simulink model "Assignment2 fake"  (R2020a)
settings: Solver=FixedStepAuto  StartTime=0.0  StopTime=10.0  FixedStep=1e-3  RelTol=1e-3  EnableMultiTasking=on
undefined symbols (not defined in the file): A0, A1, D0, D1, D10, D11, D12, D13, D2, D3, D4, D5, D6, D7, D8, D9, PTA0, PTA1, PTA2, PTB2, PTB23, PTB3, PTB9, PTC16, PTC17, PTC2, PTC3, PTC4, PTD0, PTD1, PTD2, PTD3
libraries: frdmk64flib x25, etargetslib x2
settings Model: ExtModeTrigDuration=5  Creator=theodor  LastModifiedBy=theodor
settings OptimizationCC: EnhancedBackFolding=on  PassReuseOutputArgsAs=Individual arguments  ZeroExternalMemoryAtStartup=off  ZeroInternalMemoryAtStartup=off  MaxStackSize=64  OptimizeBlockOrder=speed  DifferentSizesBufferReuse=on  OptimizationCustomize=off  EfficientTunableParamExpr=on
settings DebuggingCC: ParameterTunabilityLossMsg=error
settings HardwareCC: ProdBitPerPointer=32  ProdBitPerSizeT=32  ProdBitPerPtrDiffT=32  ProdLargestAtomicInteger=Long  ProdLargestAtomicFloat=Double  ProdWordSize=32  ProdHWDeviceType=ARM Compatible->ARM Cortex
settings SFSimCC: MATLABDynamicMemAlloc=off
settings RTWCC: SystemTargetFile=ert.tlc  HardwareBoard=NXP FRDM-K64F  TemplateMakefile=ert_default_tmf  Toolchain=GNU Tools for ARM Embedded Processors
settings CodeAppCC: ForceParamTrailComments=on  IgnoreCustomStorageClasses=off  OperatorAnnotations=on  SimulinkDataObjDesc=on  SFDataObjDesc=on  InsertBlockDesc=on

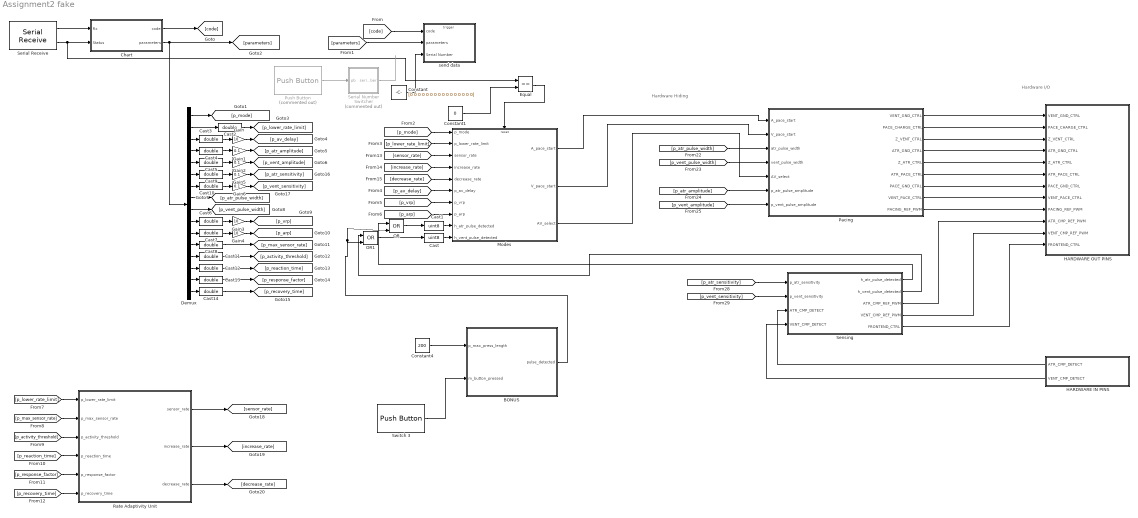
== system Assignment2 fake ==
  note: Hardware I/O
  note: Hardware Hiding
  BONUS : Stateflow chart  TreatAsAtomicUnit=on
  Cast : DataTypeConversion  OutDataTypeStr=uint8
  Cast1 : DataTypeConversion  OutDataTypeStr=uint8
  Cast{2..14} (13 alike) : DataTypeConversion  OutDataTypeStr=double
  Chart : Stateflow chart  TreatAsAtomicUnit=on
  Constant : Constant  Value=[0 0 0 0 0 0 0 0 0 0 0 0 0 0 0 0]  OutDataTypeStr=uint8
  Constant1 : Constant  Value=0
  Constant4 : Constant  Value=200
  Demux : Demux  Outputs=16
  Equal : RelationalOperator  Operator===  OutDataTypeStr=boolean  RndMeth=Simplest
  Gain : Gain  Gain=10
  Gain{1..2,5..6} (4 alike) : Gain  Gain=0.1
  Gain3 : Gain  Gain=10
  Gain4 : Gain  Gain=10
  HARDWARE IN PINS : Subsystem
  HARDWARE OUT PINS : Subsystem
  Modes : Subsystem
  OR : Logic  Operator=OR  IconShape=distinctive  AllPortsSameDT=off  OutDataTypeStr=boolean
  OR1 : Logic  Operator=OR  IconShape=distinctive  AllPortsSameDT=off  OutDataTypeStr=boolean
  Pacing : Subsystem
  Push Button : frdmk64flib/Push Button  Commented=on  Whichswitch=SW3  SampleTime1=-1
  Rate Adaptivity Unit : Subsystem
  Sensing : Subsystem
  Serial Number Switcher : Stateflow chart  Commented=on  TreatAsAtomicUnit=on
  Serial Receive : frdmk64flib/Serial Receive  SCIModule=0  Baudrate=uint32(9600)  Parity=None  StopBits=1  HardwareFlowControl=None  ByteOrder=LittleEndian  DataType=uint8  DataLength=17  BlockingMode=off  OutputStatus=on  SampleTime=-1
  Switch 3 : frdmk64flib/Push Button  Whichswitch=SW3  SampleTime1=-1
  send data : Subsystem
  wires:
  Serial Receive/2 -> Equal/1, Chart/2(Status)
  Chart/2(parameters) -> Demux/1, [parameters]
  Chart/1(code) -> [code]
  [code] -> send data/1(code)
  [parameters] -> send data/2(parameters)
  Demux/1 -> [p_mode]
  Demux/9 -> [p_vent_pulse_width]
  Serial Receive/1 -> Chart/1(Rx)
  Demux/2 -> Cast2/1
  Serial Number Switcher/1(serial_number) -> ?
  Demux/8 -> [p_atr_pulse_width]
  Push Button/1 -> Serial Number Switcher/1(pb)
  Demux/3 -> Cast3/1
  Demux/4 -> Cast4/1
  Demux/5 -> Cast5/1
  [p_mode] -> Modes/1(p_mode)
  [p_lower_rate_limit] -> Modes/2(p_lower_rate_limit)
  [p_av_delay] -> Modes/6(p_av_delay)
  [p_vrp] -> Modes/7(p_vrp)
  [p_arp] -> Modes/8(p_arp)
  [p_lower_rate_limit] -> Rate Adaptivity Unit/1(p_lower_rate_limit)
  [p_max_sensor_rate] -> Rate Adaptivity Unit/2(p_max_sensor_rate)
  [p_activity_threshold] -> Rate Adaptivity Unit/3(p_activity_threshold)
  [p_reaction_time] -> Rate Adaptivity Unit/4(p_reaction_time)
  [p_response_factor] -> Rate Adaptivity Unit/5(p_response_factor)
  [p_recovery_time] -> Rate Adaptivity Unit/6(p_recovery_time)
  Rate Adaptivity Unit/1(sensor_rate) -> [sensor_rate]
  Rate Adaptivity Unit/2(increase_rate) -> [increase_rate]
  Rate Adaptivity Unit/3(decrease_rate) -> [decrease_rate]
  [sensor_rate] -> Modes/3(sensor_rate)
  [increase_rate] -> Modes/4(increase_rate)
  [decrease_rate] -> Modes/5(decrease_rate)
  Pacing/6(ATR_PACE_CTRL) -> HARDWARE OUT PINS/6(ATR_PACE_CTRL)
  Pacing/1(VENT_GND_CTRL) -> HARDWARE OUT PINS/1(VENT_GND_CTRL)
  HARDWARE IN PINS/2(VENT_CMP_DETECT) -> Sensing/4(VENT_CMP_DETECT)
  Pacing/4(ATR_GND_CTRL) -> HARDWARE OUT PINS/4(ATR_GND_CTRL)
  [p_atr_sensitivity] -> Sensing/1(p_atr_sensitivity)
  [p_atr_amplitude] -> Pacing/6(p_atr_pulse_amplitude)
  [p_vent_sensitivity] -> Sensing/2(p_vent_sensitivity)
  Pacing/2(PACE_CHARGE_CTRL) -> HARDWARE OUT PINS/2(PACE_CHARGE_CTRL)
  Sensing/3(ATR_CMP_REF_PWM) -> HARDWARE OUT PINS/10(ATR_CMP_REF_PWM)
  [p_atr_pulse_width] -> Pacing/3(atr_pulse_width)
  Pacing/5(Z_ATR_CTRL) -> HARDWARE OUT PINS/5(Z_ATR_CTRL)
  [p_vent_amplitude] -> Pacing/7(p_vent_pulse_amplitude)
  Pacing/8(VENT_PACE_CTRL) -> HARDWARE OUT PINS/8(VENT_PACE_CTRL)
  HARDWARE IN PINS/1(ATR_CMP_DETECT) -> Sensing/3(ATR_CMP_DETECT)
  Sensing/5(FRONTEND_CTRL) -> HARDWARE OUT PINS/12(FRONTEND_CTRL)
  Pacing/9(PACING_REF_PWM) -> HARDWARE OUT PINS/9(PACING_REF_PWM)
  Sensing/4(VENT_CMP_REF_PWM) -> HARDWARE OUT PINS/11(VENT_CMP_REF_PWM)
  Pacing/7(PACE_GND_CTRL) -> HARDWARE OUT PINS/7(PACE_GND_CTRL)
  [p_vent_pulse_width] -> Pacing/4(vent_pulse_width)
  Pacing/3(Z_VENT_CTRL) -> HARDWARE OUT PINS/3(Z_VENT_CTRL)
  Modes/1(A_pace_start) -> Pacing/1(A_pace_start)
  Modes/2(V_pace_start) -> Pacing/2(V_pace_start)
  Modes/3(AV_select) -> Pacing/5(AV_select)
  Sensing/1(h_atr_pulse_detected) -> OR/1
  Sensing/2(h_vent_pulse_detected) -> OR1/1
  Switch 3/1 -> BONUS/2(m_button_pressed)
  Constant4/1 -> BONUS/1(p_max_press_length)
  OR/1 -> Cast1/1
  BONUS/1(pulse_detected) -> OR/2, OR1/2
  OR1/1 -> Cast/1
  Cast/1 -> Modes/10(h_vent_pulse_detected)
  Cast1/1 -> Modes/9(h_atr_pulse_detected)
  Cast2/1 -> [p_lower_rate_limit]
  Gain/1 -> [p_av_delay]
  Cast3/1 -> Gain/1
  Cast4/1 -> Gain1/1
  Gain1/1 -> [p_atr_amplitude]
  Gain2/1 -> [p_vent_amplitude]
  Cast5/1 -> Gain2/1
  Demux/10 -> Cast6/1
  Demux/11 -> Cast7/1
  Cast7/1 -> Gain4/1
  Cast6/1 -> Gain3/1
  Gain3/1 -> [p_vrp]
  Gain4/1 -> [p_arp]
  Demux/12 -> Cast8/1
  Cast8/1 -> [p_max_sensor_rate]
  Cast10/1 -> Gain6/1
  Cast9/1 -> Gain5/1
  Demux/6 -> Cast9/1
  Demux/7 -> Cast10/1
  Gain5/1 -> [p_atr_sensitivity]
  Gain6/1 -> [p_vent_sensitivity]
  Demux/13 -> Cast11/1
  Demux/14 -> Cast12/1
  Demux/15 -> Cast13/1
  Demux/16 -> Cast14/1
  Cast11/1 -> [p_activity_threshold]
  Cast12/1 -> [p_reaction_time]
  Cast13/1 -> [p_response_factor]
  Cast14/1 -> [p_recovery_time]
  Constant/1 -> send data/3(Serial Number)
  Constant1/1 -> Equal/2
  Equal/1 -> Modes/Reset

== system Assignment2 fake/HARDWARE IN PINS ==
  Cast : DataTypeConversion  OutDataTypeStr=uint8
  Cast1 : DataTypeConversion  OutDataTypeStr=uint8
  D0 : frdmk64flib/Digital Read  Whichpin=PTC16 (D0)  SampleTime=-1
  D1 : frdmk64flib/Digital Read  Whichpin=PTC17 (D1)  SampleTime=-1
  ATR_CMP_DETECT : Outport
  VENT_CMP_DETECT : Outport  Port=2
  wires:
  D1/1 -> Cast1/1
  D0/1 -> Cast/1
  Cast/1 -> ATR_CMP_DETECT/1
  Cast1/1 -> VENT_CMP_DETECT/1

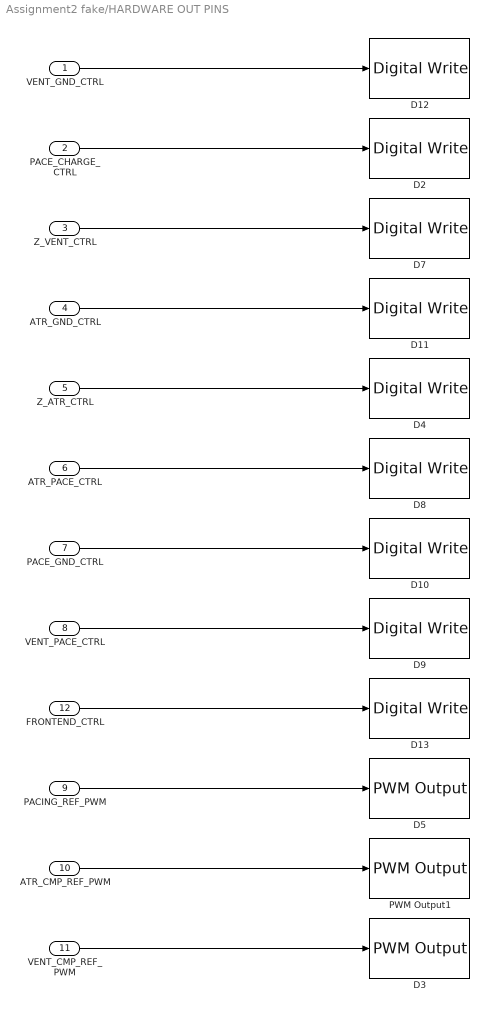
== system Assignment2 fake/HARDWARE OUT PINS ==
  VENT_GND_CTRL : Inport
  PACE_CHARGE_CTRL : Inport  Port=2
  Z_VENT_CTRL : Inport  Port=3
  ATR_GND_CTRL : Inport  Port=4
  Z_ATR_CTRL : Inport  Port=5
  ATR_PACE_CTRL : Inport  Port=6
  PACE_GND_CTRL : Inport  Port=7
  VENT_PACE_CTRL : Inport  Port=8
  PACING_REF_PWM : Inport  Port=9
  ATR_CMP_REF_PWM : Inport  Port=10
  VENT_CMP_REF_PWM : Inport  Port=11
  FRONTEND_CTRL : Inport  Port=12
  D10 : frdmk64flib/Digital Write  Whichpin=PTD0 (D10)
  D11 : frdmk64flib/Digital Write  Whichpin=PTD2 (D11)
  D12 : frdmk64flib/Digital Write  Whichpin=PTD3 (D12)
  D13 : frdmk64flib/Digital Write  Whichpin=PTD1 (D13)
  D2 : frdmk64flib/Digital Write  Whichpin=PTB9 (D2)
  D3 : frdmk64flib/PWM Output  Whichpin=PTA1 (D3)  InitialFrequency=2000  InitialDutyCycle=0
  D4 : frdmk64flib/Digital Write  Whichpin=PTB23 (D4)
  D5 : frdmk64flib/PWM Output  Whichpin=PTA2 (D5)  InitialFrequency=2000  InitialDutyCycle=0
  D7 : frdmk64flib/Digital Write  Whichpin=PTC3 (D7)
  D8 : frdmk64flib/Digital Write  Whichpin=PTA0 (D8)
  D9 : frdmk64flib/Digital Write  Whichpin=PTC4 (D9)
  PWM Output1 : frdmk64flib/PWM Output  Whichpin=PTC2 (D6)  InitialFrequency=2000  InitialDutyCycle=0
  wires:
  ATR_PACE_CTRL/1 -> D8/1
  Z_ATR_CTRL/1 -> D4/1
  VENT_GND_CTRL/1 -> D12/1
  PACE_CHARGE_CTRL/1 -> D2/1
  FRONTEND_CTRL/1 -> D13/1
  ATR_GND_CTRL/1 -> D11/1
  PACE_GND_CTRL/1 -> D10/1
  VENT_PACE_CTRL/1 -> D9/1
  Z_VENT_CTRL/1 -> D7/1
  PACING_REF_PWM/1 -> D5/1
  ATR_CMP_REF_PWM/1 -> PWM Output1/1
  VENT_CMP_REF_PWM/1 -> D3/1

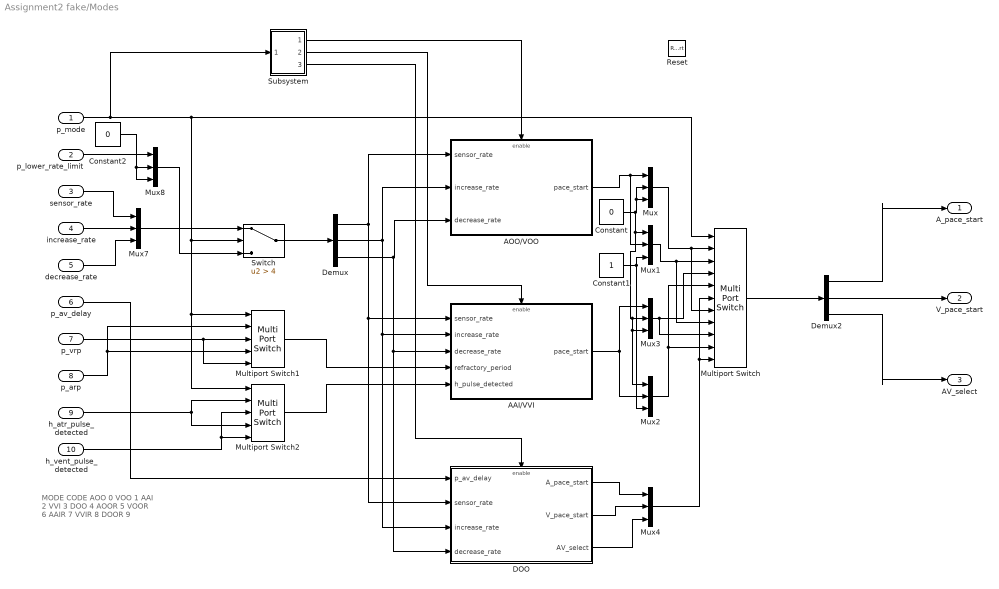
== system Assignment2 fake/Modes ==
  note: MODE
      | CODE
      |
      | AOO
      | 0
      |
      | VOO
      | 1
      |
      | AAI
      | 2
      |
      | VVI
      | 3
      |
      | DOO
      | 4
      |
      | AOOR
      | 5
      |
      | VOOR
      | 6
      |
      | AAIR
      | 7
      |
      | VVIR
      | 8
      |
      | DOOR
      | 9
  p_mode : Inport  OutDataTypeStr=uint8
  p_lower_rate_limit : Inport  Port=2
  sensor_rate : Inport  Port=3
  increase_rate : Inport  Port=4
  decrease_rate : Inport  Port=5
  p_av_delay : Inport  Port=6
  p_vrp : Inport  Port=7
  p_arp : Inport  Port=8
  h_atr_pulse_detected : Inport  Port=9
  h_vent_pulse_detected : Inport  Port=10
  Reset : ResetPort  DisableCoverage=on
  AAI/VVI : Subsystem
  AOO/VOO : Subsystem
  Constant : Constant  Value=0  OutDataTypeStr=boolean
  Constant1 : Constant  OutDataTypeStr=boolean
  Constant2 : Constant  Value=0  OutDataTypeStr=double
  DOO : Subsystem
  Demux : Demux  Outputs=3
  Demux2 : Demux  Outputs=3
  Multiport Switch : MultiPortSwitch  DataPortOrder=Zero-based contiguous  Inputs=10  zeroidx=on
  Multiport Switch1 : MultiPortSwitch  DataPortOrder=Specify indices  Inputs=10  DataPortIndices={2,3,7,8}  DiagnosticForDefault=None
  Multiport Switch2 : MultiPortSwitch  DataPortOrder=Specify indices  Inputs=10  DataPortIndices={2,3,7,8}  DiagnosticForDefault=None
  Mux{,1..4,7..8} (7 alike) : Mux  Inputs=3
  Subsystem : Subsystem
  Switch : Switch  Criteria=u2 > Threshold  Threshold=4
  A_pace_start : Outport
  V_pace_start : Outport  Port=2
  AV_select : Outport  Port=3
  wires:
  Demux2/2 -> V_pace_start/1
  Multiport Switch/1 -> Demux2/1
  Demux2/1 -> A_pace_start/1
  AOO/VOO/1(pace_start) -> Mux1/2, Mux/1
  Demux/3 -> DOO/4(decrease_rate), AAI/VVI/3(decrease_rate), AOO/VOO/3(decrease_rate)
  Demux/1 -> AOO/VOO/1(sensor_rate), DOO/2(sensor_rate), AAI/VVI/1(sensor_rate)
  Demux/2 -> DOO/3(increase_rate), AAI/VVI/2(increase_rate), AOO/VOO/2(increase_rate)
  p_av_delay/1 -> DOO/1(p_av_delay)
  Demux2/3 -> AV_select/1
  Switch/1 -> Demux/1
  Constant/1 -> Mux2/1, Mux3/3, Mux3/2, Mux1/1, Mux/3, Mux/2
  Constant1/1 -> Mux2/3, Mux1/3
  AAI/VVI/1(pace_start) -> Mux2/2, Mux3/1
  DOO/1(A_pace_start) -> Mux4/1
  DOO/2(V_pace_start) -> Mux4/2
  DOO/3(AV_select) -> Mux4/3
  Mux/1 -> Multiport Switch/7, Multiport Switch/2
  Mux1/1 -> Multiport Switch/3, Multiport Switch/8
  Mux3/1 -> Multiport Switch/9, Multiport Switch/4
  Mux2/1 -> Multiport Switch/10, Multiport Switch/5
  Mux4/1 -> Multiport Switch/11, Multiport Switch/6
  Constant2/1 -> Mux8/3, Mux8/2
  p_lower_rate_limit/1 -> Mux8/1
  sensor_rate/1 -> Mux7/1
  increase_rate/1 -> Mux7/2
  decrease_rate/1 -> Mux7/3
  Mux7/1 -> Switch/1
  Mux8/1 -> Switch/3
  p_mode/1 -> Subsystem/1(In1), Multiport Switch/1, Multiport Switch2/1, Multiport Switch1/1, Switch/2
  Subsystem/1(Out1) -> AOO/VOO/Enable
  Subsystem/2(Out2) -> AAI/VVI/Enable
  Subsystem/3(Out3) -> DOO/Enable
  p_arp/1 -> Multiport Switch1/4, Multiport Switch1/2
  p_vrp/1 -> Multiport Switch1/5, Multiport Switch1/3
  h_atr_pulse_detected/1 -> Multiport Switch2/2, Multiport Switch2/4
  h_vent_pulse_detected/1 -> Multiport Switch2/5, Multiport Switch2/3
  Multiport Switch1/1 -> AAI/VVI/4(refractory_period)
  Multiport Switch2/1 -> AAI/VVI/5(h_pulse_detected)

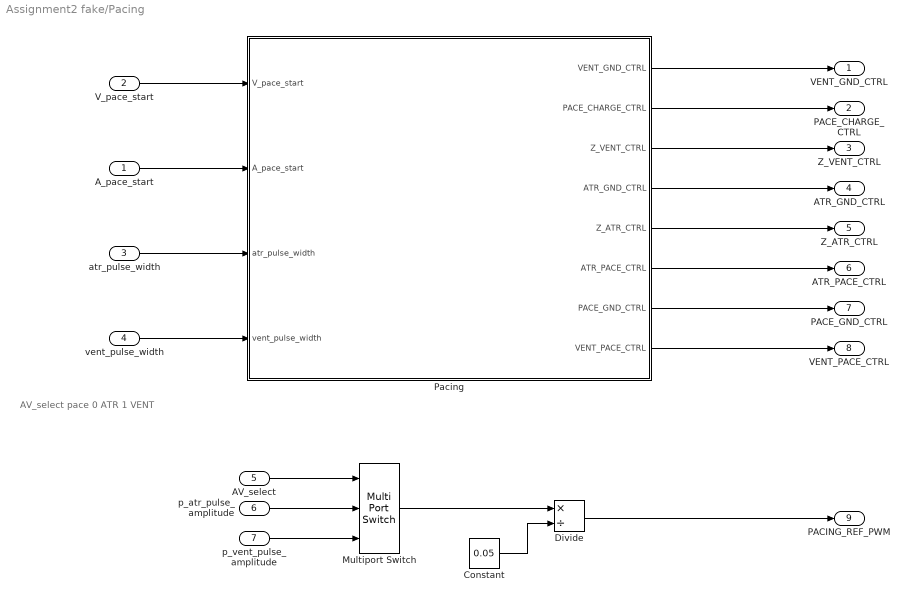
== system Assignment2 fake/Pacing ==
  note: AV_select
      | pace
      |
      | 0
      | ATR
      |
      | 1
      | VENT
  A_pace_start : Inport
  V_pace_start : Inport  Port=2
  atr_pulse_width : Inport  Port=3
  vent_pulse_width : Inport  Port=4
  AV_select : Inport  Port=5
  p_atr_pulse_amplitude : Inport  Port=6
  p_vent_pulse_amplitude : Inport  Port=7
  Constant : Constant  Value=0.05
  Divide : Product  Inputs=*/
  Multiport Switch : MultiPortSwitch  DataPortOrder=Zero-based contiguous  Inputs=2  DiagnosticForDefault=None  zeroidx=on
  Pacing : Stateflow chart  TreatAsAtomicUnit=on
  VENT_GND_CTRL : Outport
  PACE_CHARGE_CTRL : Outport  Port=2
  Z_VENT_CTRL : Outport  Port=3
  ATR_GND_CTRL : Outport  Port=4
  Z_ATR_CTRL : Outport  Port=5
  ATR_PACE_CTRL : Outport  Port=6
  PACE_GND_CTRL : Outport  Port=7
  VENT_PACE_CTRL : Outport  Port=8
  PACING_REF_PWM : Outport  Port=9
  wires:
  Pacing/3(Z_VENT_CTRL) -> Z_VENT_CTRL/1
  Pacing/6(ATR_PACE_CTRL) -> ATR_PACE_CTRL/1
  atr_pulse_width/1 -> Pacing/3(atr_pulse_width)
  A_pace_start/1 -> Pacing/2(A_pace_start)
  Pacing/5(Z_ATR_CTRL) -> Z_ATR_CTRL/1
  Pacing/2(PACE_CHARGE_CTRL) -> PACE_CHARGE_CTRL/1
  Pacing/7(PACE_GND_CTRL) -> PACE_GND_CTRL/1
  Pacing/8(VENT_PACE_CTRL) -> VENT_PACE_CTRL/1
  Pacing/4(ATR_GND_CTRL) -> ATR_GND_CTRL/1
  V_pace_start/1 -> Pacing/1(V_pace_start)
  Pacing/1(VENT_GND_CTRL) -> VENT_GND_CTRL/1
  AV_select/1 -> Multiport Switch/1
  p_atr_pulse_amplitude/1 -> Multiport Switch/2
  p_vent_pulse_amplitude/1 -> Multiport Switch/3
  Multiport Switch/1 -> Divide/1
  Constant/1 -> Divide/2
  Divide/1 -> PACING_REF_PWM/1
  vent_pulse_width/1 -> Pacing/4(vent_pulse_width)

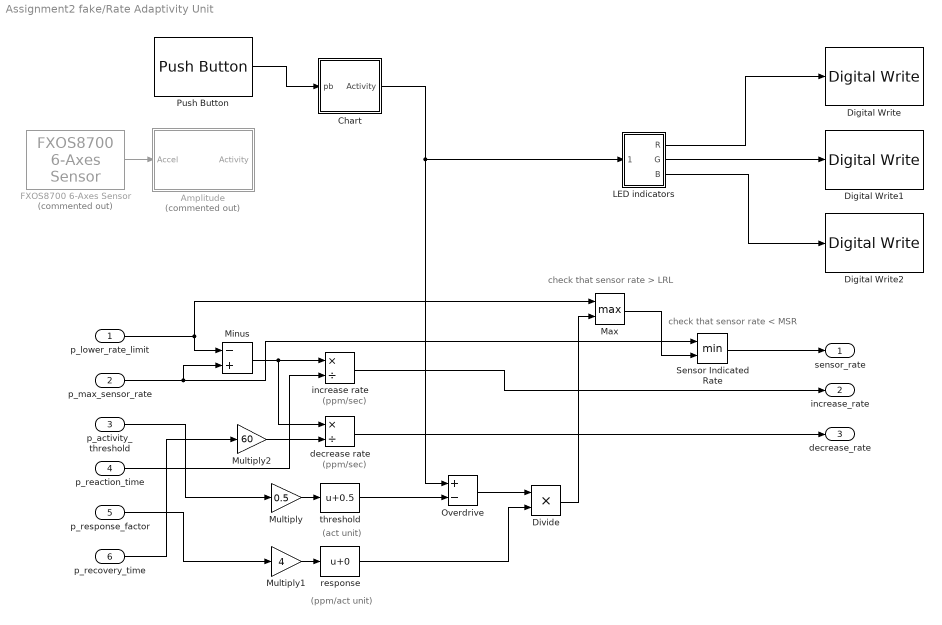
== system Assignment2 fake/Rate Adaptivity Unit ==
  note: check that sensor rate < MSR
  note: check that sensor rate > LRL
  note: (ppm/act unit)
  note: (act unit)
  note: (ppm/sec)
  note: (ppm/sec)
  p_lower_rate_limit : Inport
  p_max_sensor_rate : Inport  Port=2
  p_activity_threshold : Inport  Port=3
  p_reaction_time : Inport  Port=4
  p_response_factor : Inport  Port=5
  p_recovery_time : Inport  Port=6
  Amplitude : Subsystem  Commented=on
  Chart : Stateflow chart  TreatAsAtomicUnit=on
  Digital Write : frdmk64flib/Digital Write  Whichpin=RED_LED
  Digital Write1 : frdmk64flib/Digital Write  Whichpin=GREEN_LED
  Digital Write2 : frdmk64flib/Digital Write  Whichpin=BLUE_LED
  Divide : Product  Inputs=**
  FXOS8700 6-Axes Sensor : frdmk64flib/FXOS8700 6-Axes Sensor  Commented=on  Activesensor=Accelerometer only  ODR=100Hz  HybridODR=100Hz  Accelfullrange=-4g to +4g  SampleTime=-1
  LED indicators : Subsystem
  Max : MinMax  Function=max  Inputs=2
  Minus : Sum  Inputs=-+
  Multiply : Gain  Gain=0.5
  Multiply1 : Gain  Gain=4
  Multiply2 : Gain  Gain=60
  Overdrive : Sum  Inputs=+-
  Push Button : frdmk64flib/Push Button  Whichswitch=SW2  SampleTime1=-1
  Sensor Indicated Rate : MinMax  Inputs=2
  decrease rate : Product  Inputs=*/
  increase rate : Product  Inputs=*/
  response : Bias
  threshold : Bias  Bias=0.5
  sensor_rate : Outport
  increase_rate : Outport  Port=2
  decrease_rate : Outport  Port=3
  wires:
  FXOS8700 6-Axes Sensor/1 -> Amplitude/1(Accel)
  p_lower_rate_limit/1 -> Max/1, Minus/1
  p_max_sensor_rate/1 -> Minus/2, Sensor Indicated Rate/1
  Minus/1 -> decrease rate/1, increase rate/1
  p_reaction_time/1 -> increase rate/2
  Multiply/1 -> threshold/1
  p_activity_threshold/1 -> Multiply/1
  Multiply1/1 -> response/1
  p_response_factor/1 -> Multiply1/1
  Max/1 -> Sensor Indicated Rate/2
  threshold/1 -> Overdrive/2
  response/1 -> Divide/2
  Overdrive/1 -> Divide/1
  Divide/1 -> Max/2
  Sensor Indicated Rate/1 -> sensor_rate/1
  increase rate/1 -> increase_rate/1
  decrease rate/1 -> decrease_rate/1
  Multiply2/1 -> decrease rate/2
  p_recovery_time/1 -> Multiply2/1
  Chart/1(Activity) -> Overdrive/1, LED indicators/1(input)
  LED indicators/2(G) -> Digital Write1/1
  LED indicators/1(R) -> Digital Write/1
  LED indicators/3(B) -> Digital Write2/1
  Push Button/1 -> Chart/1(pb)

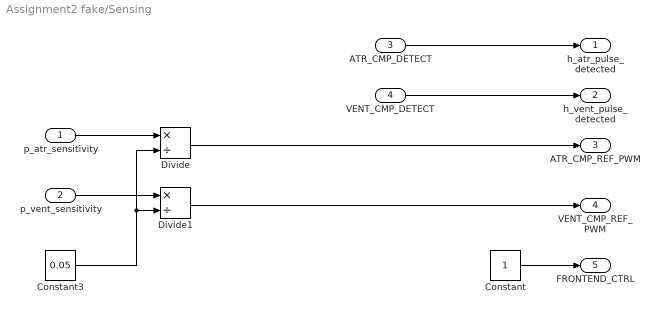
== system Assignment2 fake/Sensing ==
  p_atr_sensitivity : Inport
  p_vent_sensitivity : Inport  Port=2
  ATR_CMP_DETECT : Inport  Port=3
  VENT_CMP_DETECT : Inport  Port=4
  Constant : Constant  OutDataTypeStr=boolean
  Constant3 : Constant  Value=0.05
  Divide : Product  Inputs=*/
  Divide1 : Product  Inputs=*/
  h_atr_pulse_detected : Outport
  h_vent_pulse_detected : Outport  Port=2
  ATR_CMP_REF_PWM : Outport  Port=3
  VENT_CMP_REF_PWM : Outport  Port=4
  FRONTEND_CTRL : Outport  Port=5
  wires:
  Constant/1 -> FRONTEND_CTRL/1
  Divide/1 -> ATR_CMP_REF_PWM/1
  Divide1/1 -> VENT_CMP_REF_PWM/1
  ATR_CMP_DETECT/1 -> h_atr_pulse_detected/1
  VENT_CMP_DETECT/1 -> h_vent_pulse_detected/1
  p_atr_sensitivity/1 -> Divide/1
  p_vent_sensitivity/1 -> Divide1/1
  Constant3/1 -> Divide1/2, Divide/2

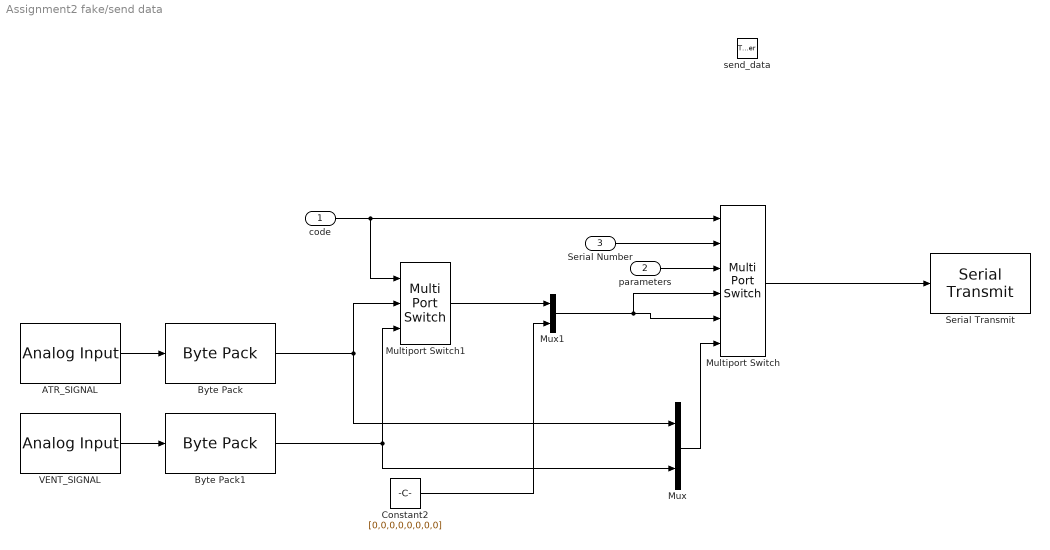
== system Assignment2 fake/send data ==
  code : Inport
  parameters : Inport  Port=2
  Serial Number : Inport  Port=3  OutDataTypeStr=uint8
  send_data : TriggerPort  TriggerType=function-call  IsSimulinkFunction=on  FunctionName=send_data  VariantControl=Variant  PortDimensions=1
  ATR_SIGNAL : frdmk64flib/Analog Input  Whichpin=PTB2 (A0)  SampleTime=-1
  Byte Pack : etargetslib/Byte Pack  datatypes={'double'}  byteAlign=1
  Byte Pack1 : etargetslib/Byte Pack  datatypes={'double'}  byteAlign=1
  Constant2 : Constant  Value=[0,0,0,0,0,0,0,0]  OutDataTypeStr=uint8
  Multiport Switch : MultiPortSwitch  DataPortOrder=Specify indices  DataPortIndices={0,2,3,4,5}  DiagnosticForDefault=None
  Multiport Switch1 : MultiPortSwitch  DataPortOrder=Specify indices  DataPortIndices={3,4}  DiagnosticForDefault=None
  Mux : Mux  Inputs=2
  Mux1 : Mux  Inputs=2
  Serial Transmit : frdmk64flib/Serial Transmit  SCIModule=0  Baudrate=uint32(9600)  Parity=None  StopBits=1  HardwareFlowControl=None  ByteOrder=LittleEndian  BlockingMode=on  OutputStatus=off
  VENT_SIGNAL : frdmk64flib/Analog Input  Whichpin=PTB3 (A1)  SampleTime=-1
  wires:
  ATR_SIGNAL/1 -> Byte Pack/1
  VENT_SIGNAL/1 -> Byte Pack1/1
  code/1 -> Multiport Switch1/1, Multiport Switch/1
  Byte Pack/1 -> Multiport Switch1/2, Mux/1
  Byte Pack1/1 -> Multiport Switch1/3, Mux/2
  Mux/1 -> Multiport Switch/6
  Multiport Switch/1 -> Serial Transmit/1
  Mux1/1 -> Multiport Switch/5, Multiport Switch/4
  Constant2/1 -> Mux1/2
  Multiport Switch1/1 -> Mux1/1
  parameters/1 -> Multiport Switch/3
  Serial Number/1 -> Multiport Switch/2

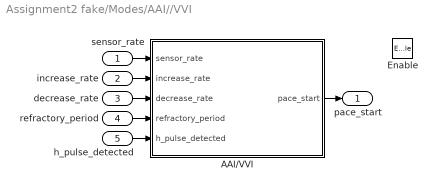
== system Assignment2 fake/Modes/AAI//VVI ==
  sensor_rate : Inport
  increase_rate : Inport  Port=2
  decrease_rate : Inport  Port=3
  refractory_period : Inport  Port=4
  h_pulse_detected : Inport  Port=5
  Enable : EnablePort  StatesWhenEnabling=reset
  AAI/VVI : Stateflow chart  TreatAsAtomicUnit=on
  pace_start : Outport
  wires:
  increase_rate/1 -> AAI/VVI/2(increase_rate)
  AAI/VVI/1(pace_start) -> pace_start/1
  refractory_period/1 -> AAI/VVI/4(refractory_period)
  h_pulse_detected/1 -> AAI/VVI/5(h_pulse_detected)
  sensor_rate/1 -> AAI/VVI/1(sensor_rate)
  decrease_rate/1 -> AAI/VVI/3(decrease_rate)

== system Assignment2 fake/Modes/AOO//VOO ==
  sensor_rate : Inport
  increase_rate : Inport  Port=2
  decrease_rate : Inport  Port=3
  Enable : EnablePort  StatesWhenEnabling=reset
  AOOR/VOOR : Stateflow chart  TreatAsAtomicUnit=on
  pace_start : Outport
  wires:
  increase_rate/1 -> AOOR/VOOR/2(increase_rate)
  decrease_rate/1 -> AOOR/VOOR/3(decrease_rate)
  sensor_rate/1 -> AOOR/VOOR/1(sensor_rate)
  AOOR/VOOR/1(pace_start) -> pace_start/1

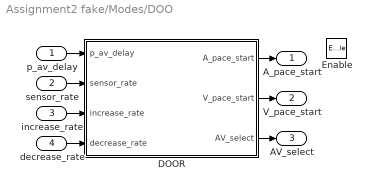
== system Assignment2 fake/Modes/DOO ==
  p_av_delay : Inport
  sensor_rate : Inport  Port=2
  increase_rate : Inport  Port=3
  decrease_rate : Inport  Port=4
  Enable : EnablePort  StatesWhenEnabling=reset
  DOOR : Stateflow chart  TreatAsAtomicUnit=on
  A_pace_start : Outport
  V_pace_start : Outport  Port=2
  AV_select : Outport  Port=3
  wires:
  decrease_rate/1 -> DOOR/4(decrease_rate)
  DOOR/3(AV_select) -> AV_select/1
  p_av_delay/1 -> DOOR/1(p_av_delay)
  increase_rate/1 -> DOOR/3(increase_rate)
  DOOR/2(V_pace_start) -> V_pace_start/1
  DOOR/1(A_pace_start) -> A_pace_start/1
  sensor_rate/1 -> DOOR/2(sensor_rate)

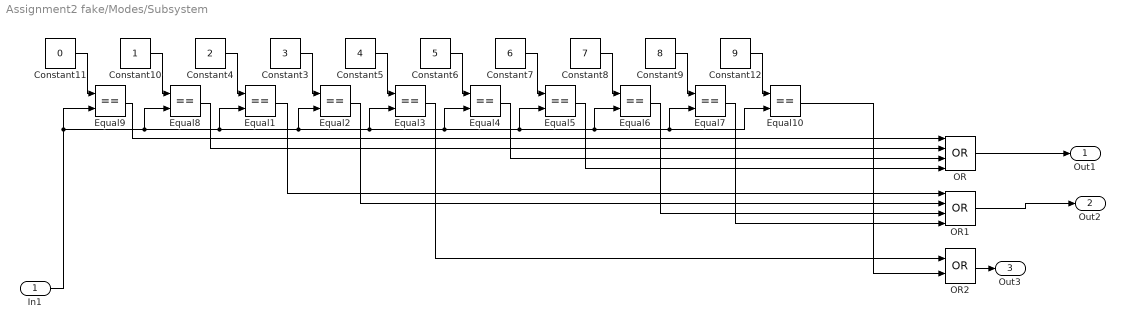
== system Assignment2 fake/Modes/Subsystem ==
  In1 : Inport
  Constant10 : Constant  OutDataTypeStr=uint8
  Constant11 : Constant  Value=0  OutDataTypeStr=uint8
  Constant12 : Constant  Value=9  OutDataTypeStr=uint8
  Constant3 : Constant  Value=3  OutDataTypeStr=uint8
  Constant4 : Constant  Value=2  OutDataTypeStr=uint8
  Constant5 : Constant  Value=4  OutDataTypeStr=uint8
  Constant6 : Constant  Value=5  OutDataTypeStr=uint8
  Constant7 : Constant  Value=6  OutDataTypeStr=uint8
  Constant8 : Constant  Value=7  OutDataTypeStr=uint8
  Constant9 : Constant  Value=8  OutDataTypeStr=uint8
  Equal{1..10} (10 alike) : RelationalOperator  Operator===  OutDataTypeStr=boolean  RndMeth=Simplest
  OR : Logic  Operator=OR  Inputs=4  AllPortsSameDT=off  OutDataTypeStr=boolean
  OR1 : Logic  Operator=OR  Inputs=4  AllPortsSameDT=off  OutDataTypeStr=boolean
  OR2 : Logic  Operator=OR  AllPortsSameDT=off  OutDataTypeStr=boolean
  Out1 : Outport
  Out2 : Outport  Port=2
  Out3 : Outport  Port=3
  wires:
  OR/1 -> Out1/1
  OR1/1 -> Out2/1
  Constant8/1 -> Equal6/1
  Constant5/1 -> Equal3/1
  OR2/1 -> Out3/1
  Equal4/1 -> OR/3
  Constant11/1 -> Equal9/1
  Equal3/1 -> OR2/1
  Constant4/1 -> Equal1/1
  Constant6/1 -> Equal4/1
  Equal7/1 -> OR1/4
  Constant3/1 -> Equal2/1
  Equal6/1 -> OR1/3
  Equal1/1 -> OR1/1
  Constant10/1 -> Equal8/1
  Equal5/1 -> OR/4
  Equal8/1 -> OR/2
  Equal9/1 -> OR/1
  Equal2/1 -> OR1/2
  Equal10/1 -> OR2/2
  Constant12/1 -> Equal10/1
  In1/1 -> Equal10/2, Equal7/2, Equal6/2, Equal5/2, Equal4/2, Equal3/2, Equal2/2, Equal1/2, Equal8/2, Equal9/2
  Constant7/1 -> Equal5/1
  Constant9/1 -> Equal7/1

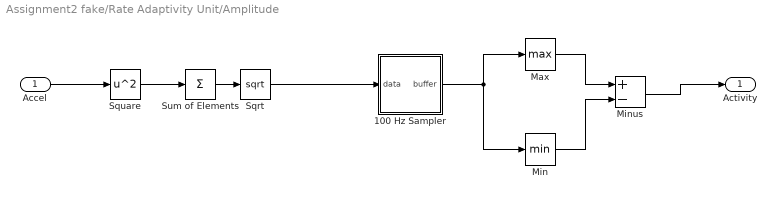
== system Assignment2 fake/Rate Adaptivity Unit/Amplitude ==
  Accel : Inport
  100 Hz Sampler : Stateflow chart  TreatAsAtomicUnit=on
  Max : MinMax  Function=max
  Min : MinMax
  Minus : Sum  Inputs=+-
  Sqrt : Sqrt  SaturateOnIntegerOverflow=on
  Square : Math  Operator=square  SaturateOnIntegerOverflow=on
  Sum of Elements : Sum  Inputs=+
  Activity : Outport
  wires:
  Accel/1 -> Square/1
  Square/1 -> Sum of Elements/1
  Sum of Elements/1 -> Sqrt/1
  Sqrt/1 -> 100 Hz Sampler/1(data)
  100 Hz Sampler/1(buffer) -> Max/1, Min/1
  Max/1 -> Minus/1
  Min/1 -> Minus/2
  Minus/1 -> Activity/1

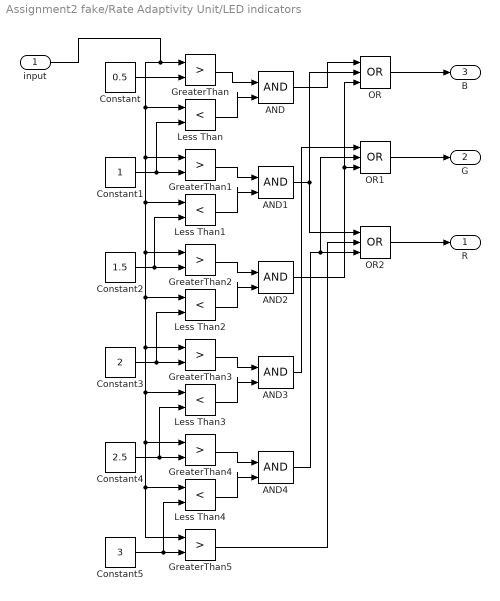
== system Assignment2 fake/Rate Adaptivity Unit/LED indicators ==
  input : Inport
  AND{,1..4} (5 alike) : Logic  IconShape=distinctive  AllPortsSameDT=off  OutDataTypeStr=boolean
  Constant : Constant  Value=0.5
  Constant1 : Constant
  Constant2 : Constant  Value=1.5
  Constant3 : Constant  Value=2
  Constant4 : Constant  Value=2.5
  Constant5 : Constant  Value=3
  GreaterThan{,1..5} (6 alike) : RelationalOperator  Operator=>  OutDataTypeStr=boolean  RndMeth=Simplest
  Less Than{,1..4} (5 alike) : RelationalOperator  Operator=<  OutDataTypeStr=boolean  RndMeth=Simplest
  OR : Logic  Operator=OR  Inputs=3  IconShape=distinctive  AllPortsSameDT=off  OutDataTypeStr=boolean
  OR1 : Logic  Operator=OR  Inputs=3  IconShape=distinctive  AllPortsSameDT=off  OutDataTypeStr=boolean
  OR2 : Logic  Operator=OR  Inputs=3  IconShape=distinctive  AllPortsSameDT=off  OutDataTypeStr=boolean
  R : Outport
  G : Outport  Port=2
  B : Outport  Port=3
  wires:
  OR1/1 -> G/1
  Less Than4/1 -> AND4/2
  Less Than/1 -> AND/2
  Constant/1 -> GreaterThan/2
  AND1/1 -> OR2/1, OR/2
  OR/1 -> B/1
  AND4/1 -> OR1/2, OR2/3
  GreaterThan1/1 -> AND1/1
  Less Than3/1 -> AND3/2
  OR2/1 -> R/1
  AND/1 -> OR/1
  Constant2/1 -> Less Than1/2, GreaterThan2/2
  AND3/1 -> OR1/1
  GreaterThan5/1 -> OR2/2
  Constant5/1 -> Less Than4/2, GreaterThan5/2
  Constant1/1 -> Less Than/2, GreaterThan1/2
  input/1 -> GreaterThan/1, Less Than/1, GreaterThan1/1, Less Than1/1, GreaterThan2/1, Less Than2/1, GreaterThan3/1, Less Than3/1, GreaterThan4/1, Less Than4/1, GreaterThan5/1
  GreaterThan3/1 -> AND3/1
  GreaterThan2/1 -> AND2/1
  GreaterThan/1 -> AND/1
  Less Than2/1 -> AND2/2
  AND2/1 -> OR1/3, OR/3
  Less Than1/1 -> AND1/2
  Constant4/1 -> Less Than3/2, GreaterThan4/2
  Constant3/1 -> Less Than2/2, GreaterThan3/2
  GreaterThan4/1 -> AND4/1

== stateflow chart Assignment2 fake/Modes/AAI//VVI/AAI//VVI ==
  state INITIAL
    entry:
    current_LRL = sensor_rate;
    exit:
    t = elapsed(sec);
  state SENSE
    exit:
    t = t + elapsed(sec);
  state WAIT
    exit:
    t = elapsed(sec)
  state PACE
    entry:
    pace_start = true;
    on after(1, msec):
    pace_start = false;
    exit:
    t = t + elapsed(sec);
  (default) -> INITIAL
  INITIAL -> SENSE [order 2] : [h_pulse_detected == 1]
  INITIAL -> PACE [order 1] : after(60/current_LRL, sec)
  (junction 35) -> (junction 37)
  (junction 37) -> (junction 32)
  (junction 13) -> (junction 35) [order 1] : [current_LRL + increase_rate*t > sensor_rate]{current_LRL = sensor_rate}
  (junction 13) -> (junction 32) [order 2] : {current_LRL = current_LRL + increase_rate*t}
  (junction 32) -> WAIT
  (junction 42) -> (junction 13) [order 2] : [sensor_rate > current_LRL]
  SENSE -> (junction 49)
  WAIT -> SENSE [order 2] : [h_pulse_detected == 1]
  PACE -> (junction 49)
  (junction 49) -> (junction 42) : after(refractory_period, msec)
  (junction 42) -> (junction 14) [order 1] : [sensor_rate <= current_LRL]
  WAIT -> PACE [order 1] : after(60/current_LRL - refractory_period/1000 + 0.001,sec)
  (junction 24) -> WAIT
  (junction 14) -> (junction 24) [order 2] : {current_LRL = current_LRL - decrease_rate * t}
  (junction 29) -> (junction 24)
  (junction 14) -> (junction 26) [order 1] : [current_LRL - decrease_rate * t  < sensor_rate ]{current_LRL = sensor_rate}
  (junction 26) -> (junction 29)
  data: pace_start output =false; sensor_rate input; increase_rate input; decrease_rate input; current_LRL local; t local =0; refractory_period input; h_pulse_detected input

== stateflow chart Assignment2 fake/Modes/DOO/DOOR ==
  state INITIAL
    entry:
    current_LRL = sensor_rate;
  state PACE_VENT
    entry:
    V_pace_start = true;
    on after(1, msec):
    V_pace_start = false;
    AV_select = false;
    exit:
    t = elapsed(sec)
  state PACE_ATR
    entry:
    A_pace_start = true;
    on after(1,msec):
    A_pace_start = false;
    AV_select = true;
    exit:
    t = t + elapsed(sec)
  (default) -> INITIAL
  INITIAL -> PACE_VENT
  (junction 35) -> (junction 37)
  (junction 37) -> (junction 32)
  (junction 13) -> (junction 35) [order 1] : [current_LRL + increase_rate*t > sensor_rate]{current_LRL = sensor_rate}
  (junction 13) -> (junction 32) [order 2] : {current_LRL = current_LRL + increase_rate*t}
  (junction 32) -> PACE_VENT
  (junction 42) -> (junction 13) [order 2] : [sensor_rate > current_LRL]
  PACE_ATR -> (junction 42) : after(p_av_delay, msec)
  (junction 42) -> (junction 14) [order 1] : [sensor_rate <= current_LRL]
  PACE_VENT -> PACE_ATR : after(60/current_LRL - p_av_delay/1000,sec)
  (junction 24) -> PACE_VENT
  (junction 14) -> (junction 24) [order 2] : {current_LRL = current_LRL - decrease_rate * t}
  (junction 29) -> (junction 24)
  (junction 14) -> (junction 26) [order 1] : [current_LRL - decrease_rate * t  < sensor_rate ]{current_LRL = sensor_rate}
  (junction 26) -> (junction 29)
  data: p_av_delay input; A_pace_start output =false; V_pace_start output =false; sensor_rate input; increase_rate input; decrease_rate input; current_LRL local; t local =0; AV_select output boolean

== stateflow chart Assignment2 fake/Chart ==
  state SEND_DATA
    entry:
    code = Rx(1);
    send_data();
  state INITIAL
    parameters = uint8([0 60 15 35 35 35 35 5 5 32 25 120 3 30 8 5]')
  state IDLE
  state READ_DATA
    entry:
    code = 1;
    parameters = Rx(2:17);
  (junction 39) -> (junction 41)
  (junction 41) -> IDLE : [Status==32]
  (junction 36) -> (junction 39)
  (default) -> INITIAL
  (junction 27) -> SEND_DATA [order 2]
  SEND_DATA -> (junction 36)
  INITIAL -> IDLE
  IDLE -> (junction 27) : [Status == 0]
  (junction 27) -> READ_DATA [order 1] : [Rx(1)==1]
  READ_DATA -> (junction 36)
  data: code output uint8; Rx input uint8 size=17; Status input uint8; parameters output uint8 size=16

== stateflow chart Assignment2 fake/Serial Number Switcher ==
  state S_0
    entry:
    serial_number = uint8([108 97 98 49 45 103 114 111 117 112 56 45 49 48 48 37]');
  state BUF_0
  state S_1
    entry:
    serial_number = uint8([112 97 99 101 109 97 107 101 114 98 114 101 97 107 101 114]');
  state BUF_1
  (default) -> S_0
  BUF_0 -> S_1 : [pb==1]
  S_0 -> BUF_0 : [pb==0]
  BUF_1 -> S_0 : [pb==1]
  S_1 -> BUF_1 : [pb==0]
  data: pb input; serial_number output size=16

== stateflow chart Assignment2 fake/Rate Adaptivity Unit/Amplitude/100 Hz Sampler ==
  state SAMPLE
    entry:
    buffer(2:25) = buffer(1:24);
    buffer(1) = data;
  (default) -> SAMPLE
  SAMPLE -> SAMPLE : after(40,msec)
  data: data input; buffer output size=25 =zeros(25,1)

== stateflow chart Assignment2 fake/BONUS ==
  state INVALID_PULSE
  note: buffer to ensure one button press doesn't trigger cycles
  state IDLE
    entry:
    pulse_detected = 0;
  state BUTTON_DOWN
    exit:
  note: if button is held for longer than
      | what is defined as a "quick press"
  note: buffer to ensure one button
      | press doesn't trigger cycles
  state VALID_PULSE
    entry:
    pulse_detected = 1;
  note: 1 ms pulse on pulse_detected
  INVALID_PULSE -> IDLE : [~m_button_pressed]
  BUTTON_DOWN -> INVALID_PULSE [order 2] : after(p_max_press_length,msec)
  (default) -> IDLE
  IDLE -> BUTTON_DOWN : [m_button_pressed]
  VALID_PULSE -> IDLE : after(1,msec)
  BUTTON_DOWN -> VALID_PULSE [order 1] : [~m_button_pressed]
  data: p_max_press_length input; pulse_detected output uint8; m_button_pressed input boolean

== stateflow chart Assignment2 fake/Pacing/Pacing ==
  state Buffer
  state A_Pacing
    entry:
    PACE_CHARGE_CTRL=false;
    VENT_PACE_CTRL=false;
    VENT_GND_CTRL=false;
    ATR_GND_CTRL=false;
    ATR_PACE_CTRL=true;
  state V_Pacing
    entry:
    PACE_CHARGE_CTRL=false;
    ATR_PACE_CTRL=false;
    ATR_GND_CTRL=false;
    VENT_GND_CTRL=false;
    VENT_PACE_CTRL=true;
  state INITIAL
    entry:
    VENT_GND_CTRL=false;
    Z_VENT_CTRL=false;
    Z_ATR_CTRL=false;
    ATR_GND_CTRL=false;
  state C22_Charge
    entry:
    VENT_PACE_CTRL=false;
    ATR_PACE_CTRL=false;
    PACE_CHARGE_CTRL=true;
    PACE_GND_CTRL=true;
  state C21_Discharge_V
    entry:
    VENT_PACE_CTRL=false;
    VENT_GND_CTRL=true;
  state C21_Discharge_A
    entry:
    ATR_PACE_CTRL=false;
    ATR_GND_CTRL=true;
  Buffer -> V_Pacing [order 1] : [V_pace_start==true]
  Buffer -> A_Pacing [order 2] : [A_pace_start==true]
  C22_Charge -> Buffer : [V_pace_start==false && A_pace_start==false]
  (default) -> INITIAL
  INITIAL -> C22_Charge
  C21_Discharge_A -> C22_Charge
  C21_Discharge_V -> C22_Charge
  A_Pacing -> C21_Discharge_A : after(atr_pulse_width,msec)
  V_Pacing -> C21_Discharge_V : after(vent_pulse_width,msec)
  data: VENT_GND_CTRL output boolean; PACE_CHARGE_CTRL output boolean; Z_VENT_CTRL output boolean; ATR_GND_CTRL output boolean; Z_ATR_CTRL output boolean; ATR_PACE_CTRL output boolean; PACE_GND_CTRL output boolean; VENT_PACE_CTRL output boolean; V_pace_start input boolean; A_pace_start input boolean; atr_pulse_width input; vent_pulse_width input

== stateflow chart Assignment2 fake/Rate Adaptivity Unit/Chart ==
  state ON
    entry:
    Activity = 4;
  state OFF
    entry:
    Activity = 0;
  (default) -> OFF
  OFF -> ON : [pb == 1]
  ON -> OFF : [pb == 0]
  data: pb input; Activity output

== stateflow chart Assignment2 fake/Modes/AOO//VOO/AOOR//VOOR ==
  state INITIAL
    entry:
    current_LRL = sensor_rate;
  state UPDATE_RATE
    on after(1,msec):
    pace_start = false;
    exit:
    t = elapsed(sec)
  state PACE
    entry:
    pace_start = true;
  (default) -> INITIAL
  INITIAL -> PACE
  (junction 35) -> (junction 37)
  (junction 37) -> (junction 32)
  (junction 13) -> (junction 35) [order 1] : [current_LRL + increase_rate*t > sensor_rate]{current_LRL = sensor_rate}
  (junction 13) -> (junction 32) [order 2] : {current_LRL = current_LRL + increase_rate*t}
  (junction 32) -> UPDATE_RATE
  (junction 42) -> (junction 13) [order 2] : [sensor_rate > current_LRL]
  PACE -> (junction 42)
  (junction 42) -> (junction 14) [order 1] : [sensor_rate <= current_LRL]
  UPDATE_RATE -> PACE : after(60/current_LRL,sec)
  (junction 24) -> UPDATE_RATE
  (junction 14) -> (junction 24) [order 2] : {current_LRL = current_LRL - decrease_rate * t}
  (junction 29) -> (junction 24)
  (junction 14) -> (junction 26) [order 1] : [current_LRL - decrease_rate * t  < sensor_rate ]{current_LRL = sensor_rate}
  (junction 26) -> (junction 29)
  data: pace_start output =false; sensor_rate input; increase_rate input; decrease_rate input; current_LRL local; t local =0
